simulink model "simu"  (R2023a)
settings: Solver=VariableStepAuto  StartTime=0.0  StopTime=5  RelTol=1e-3
settings Model: Creator=1  LastModifiedBy=liukan
settings DebuggingCC: UnconnectedInputMsg=warning  UnconnectedOutputMsg=warning  UnconnectedLineMsg=warning
settings ModelReferenceCC: EnableRefExpFcnMdlSchedulingChecks=on
settings RTWCC: DLArmComputeVersion=19.05

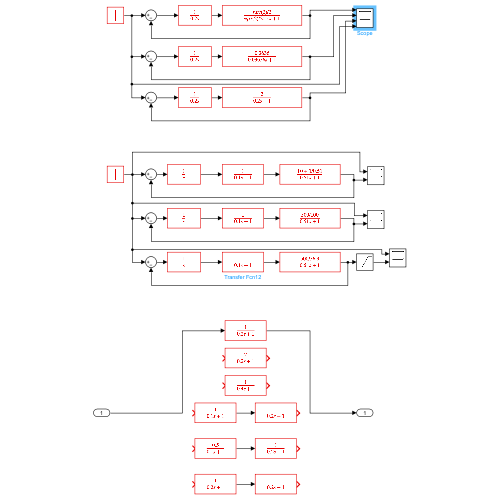
[thumbnail: Simulink's stored preview of the top-level diagram]
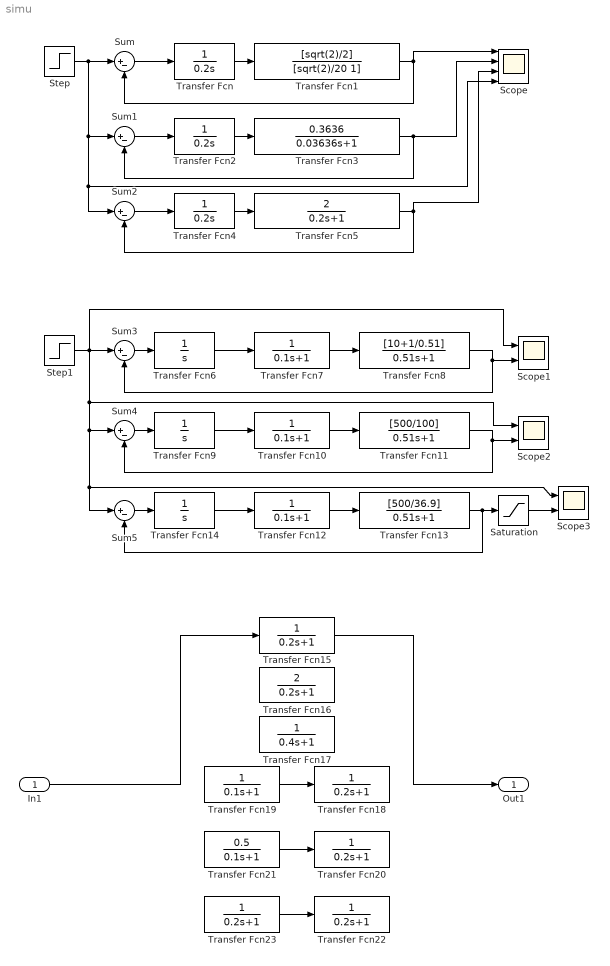
== system simu ==
  In1 : Inport
  Saturation : Saturate  UpperLimit=9  LowerLimit=-100
  Scope : Scope  NumInputPorts=4
  Scope1 : Scope  NumInputPorts=2
  Scope2 : Scope  NumInputPorts=2
  Scope3 : Scope  NumInputPorts=2
  Step : Step  After=5  SampleTime=0
  Step1 : Step  After=5  SampleTime=0
  Sum{,1..5} (6 alike) : Sum  Inputs=|+-
  Transfer Fcn : TransferFcn  Denominator=[0.2 0]
  Transfer Fcn1 : TransferFcn  Numerator=[sqrt(2)/2]  Denominator=[sqrt(2)/20 1]
  Transfer Fcn{7,10,12,19} (4 alike) : TransferFcn  Denominator=[0.1 1]
  Transfer Fcn11 : TransferFcn  Numerator=[500/100]  Denominator=[0.51 1]
  Transfer Fcn13 : TransferFcn  Numerator=[500/36.9]  Denominator=[0.51 1]
  Transfer Fcn14 : TransferFcn  Denominator=[1 0]
  Transfer Fcn{15,18,20,22..23} (5 alike) : TransferFcn  Denominator=[0.2 1]
  Transfer Fcn16 : TransferFcn  Numerator=[2]  Denominator=[0.2 1]
  Transfer Fcn17 : TransferFcn  Denominator=[0.4 1]
  Transfer Fcn2 : TransferFcn  Denominator=[0.2 0]
  Transfer Fcn21 : TransferFcn  Numerator=[0.5]  Denominator=[0.1 1]
  Transfer Fcn3 : TransferFcn  Numerator=[0.3636]  Denominator=[0.03636 1]
  Transfer Fcn4 : TransferFcn  Denominator=[0.2 0]
  Transfer Fcn5 : TransferFcn  Numerator=[2]  Denominator=[0.2 1]
  Transfer Fcn6 : TransferFcn  Denominator=[1 0]
  Transfer Fcn8 : TransferFcn  Numerator=[10+1/0.51]  Denominator=[0.51 1]
  Transfer Fcn9 : TransferFcn  Denominator=[1 0]
  Out1 : Outport
  wires:
  Transfer Fcn/1 -> Transfer Fcn1/1
  Transfer Fcn1/1 -> Scope/1, Sum/2
  Step/1 -> Sum2/1, Scope/4, Sum1/1, Sum/1
  Sum/1 -> Transfer Fcn/1
  Transfer Fcn2/1 -> Transfer Fcn3/1
  Transfer Fcn3/1 -> Scope/2, Sum1/2
  Sum1/1 -> Transfer Fcn2/1
  Transfer Fcn4/1 -> Transfer Fcn5/1
  Transfer Fcn5/1 -> Scope/3, Sum2/2
  Sum2/1 -> Transfer Fcn4/1
  Transfer Fcn6/1 -> Transfer Fcn7/1
  Step1/1 -> Scope3/1, Sum5/1, Sum4/1, Scope2/1, Scope1/1, Sum3/1
  Sum3/1 -> Transfer Fcn6/1
  Transfer Fcn7/1 -> Transfer Fcn8/1
  Transfer Fcn8/1 -> Scope1/2, Sum3/2
  Transfer Fcn11/1 -> Scope2/2, Sum4/2
  Transfer Fcn10/1 -> Transfer Fcn11/1
  Sum4/1 -> Transfer Fcn9/1
  Transfer Fcn9/1 -> Transfer Fcn10/1
  Transfer Fcn14/1 -> Transfer Fcn12/1
  Transfer Fcn12/1 -> Transfer Fcn13/1
  Sum5/1 -> Transfer Fcn14/1
  Transfer Fcn13/1 -> Sum5/2, Saturation/1
  Saturation/1 -> Scope3/2
  Transfer Fcn19/1 -> Transfer Fcn18/1
  Transfer Fcn21/1 -> Transfer Fcn20/1
  Transfer Fcn23/1 -> Transfer Fcn22/1
  In1/1 -> Transfer Fcn15/1
  Transfer Fcn15/1 -> Out1/1
